simulink model "Tra_Grip"  (R2016b)
settings: configuration reference "CodeGenConfigSet" (kept outside this file)
values from neighbouring files (symbols this model uses):
  GEAR0 = fi(0,Tra_num)    [init_Tra_Grip.m]
settings Model: Creator=Colin  LastModifiedBy=Colin
settings ConfigSetRef: SourceLocation=Base Workspace

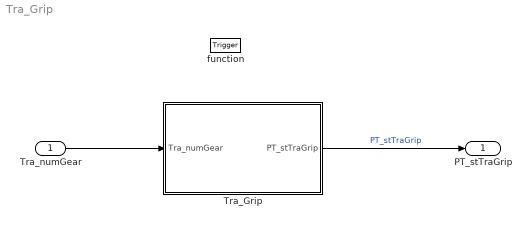
== system Tra_Grip ==
  Tra_numGear : Inport  Description=Current gear information  OutMin=-128  OutMax=127  OutDataTypeStr=Tra_num
  function : TriggerPort  TriggerType=function-call  VariantControl=Variant
  Tra_Grip : Subsystem
  PT_stTraGrip : Outport  Description=Gearbox grip status  OutMin=0  OutMax=1  OutDataTypeStr=boolean
  wires:
  Tra_Grip/1(PT_stTraGrip) -> PT_stTraGrip/1  "PT_stTraGrip"
  Tra_numGear/1 -> Tra_Grip/1(Tra_numGear)

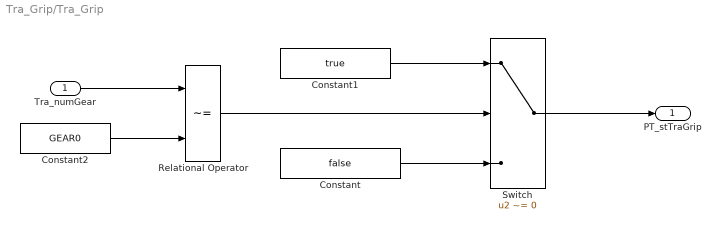
== system Tra_Grip/Tra_Grip ==
  Tra_numGear : Inport  Description=Current gear information  OutMin=-128  OutMax=127  OutDataTypeStr=Tra_num
  Constant : Constant  Value=false
  Constant1 : Constant  Value=true
  Constant2 : Constant  Value=GEAR0
  Relational Operator : RelationalOperator  Operator=~=  OutDataTypeStr=boolean  RndMeth=Simplest
  Switch : Switch  Criteria=u2 ~= 0
  PT_stTraGrip : Outport  Description=Gearbox grip status
  wires:
  Tra_numGear/1 -> Relational Operator/1
  Constant2/1 -> Relational Operator/2
  Constant1/1 -> Switch/1
  Constant/1 -> Switch/3
  Relational Operator/1 -> Switch/2
  Switch/1 -> PT_stTraGrip/1
